simulink model "berechnungVonP"  (R2016b)
settings: Solver=VariableStepAuto  StartTime=0.0  StopTime=10.0  RelTol=1e-3
undefined symbols (not defined in the file): A_ss, P_t_0, Q, R
settings Model: Creator=labor09  LastModifiedBy=labor09

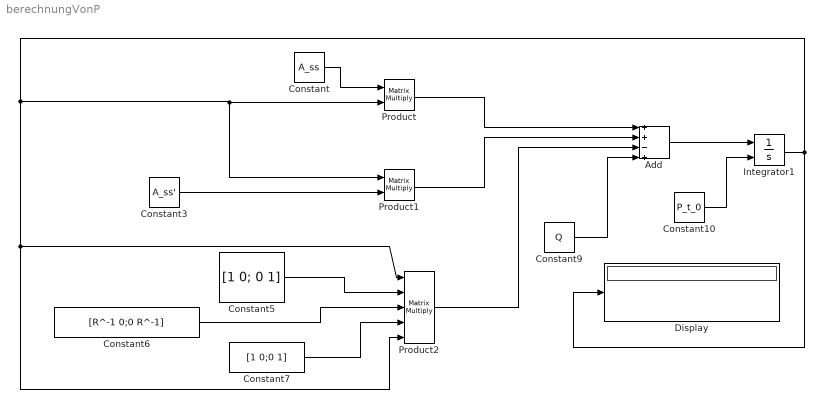
== system berechnungVonP ==
  Add : Sum  Inputs=++-+
  Constant : Constant  Value=A_ss
  Constant10 : Constant  Value=P_t_0
  Constant3 : Constant  Value=A_ss'
  Constant5 : Constant  Value=[1 0; 0 1]
  Constant6 : Constant  Value=[R^-1 0;0 R^-1]
  Constant7 : Constant  Value=[1 0;0 1]
  Constant9 : Constant  Value=Q
  Display : Display
  Integrator1 : Integrator  InitialConditionSource=external
  Product : Product  Multiplication=Matrix(*)
  Product1 : Product  Multiplication=Matrix(*)
  Product2 : Product  Inputs=5  Multiplication=Matrix(*)
  wires:
  Constant/1 -> Product/1
  Constant3/1 -> Product1/2
  Product/1 -> Add/1
  Product1/1 -> Add/2
  Constant5/1 -> Product2/2
  Product2/1 -> Add/3
  Constant9/1 -> Add/4
  Constant6/1 -> Product2/3
  Constant7/1 -> Product2/4
  Integrator1/1 -> Product2/5, Product2/1, Product/2, Product1/1, Display/1
  Add/1 -> Integrator1/1
  Constant10/1 -> Integrator1/2
